simulink model "mvdc_estimation_preprocessing"  (R2018b)
settings: configuration reference "Active" (kept outside this file)
undefined symbols (not defined in the file): P_MLOC_Loc1DelayCompTime_s, P_MLOC_Loc2DelayCompTime_s, P_MLOC_OdometryManualReset_psi_rad, P_MLOC_OdometryManualReset_x_m, P_MLOC_OdometryManualReset_y_m, P_MLOC_OdometryResetMode, P_VDC_ActivateOnlineDiagnosis, P_VDC_EnableSensorsForFusion, P_VDC_SensorFailuresLatched, psi_YawAngleLoc1_rad, psi_YawAngleLoc2_rad, tS, TUMHealthStatus, TUMStateEstimationState, tw_front_m, tw_rear_m, tyreradius_front_m, tyreradius_rear_m, valid_IMU1_b, valid_IMU2_b, valid_Loc1_b, valid_Loc2_b, valid_Vel1_b, valid_Vel2_b, x_Loc1_m, x_Loc2_m, y_Loc1_m, y_Loc2_m
libraries: simulink x10, misc x6
settings Model: DataDictionary=mvdc_estimation_preprocessing.sldd  OrderedModelArguments=off  Creator=wischnewski  LastModifiedBy=ge34qer

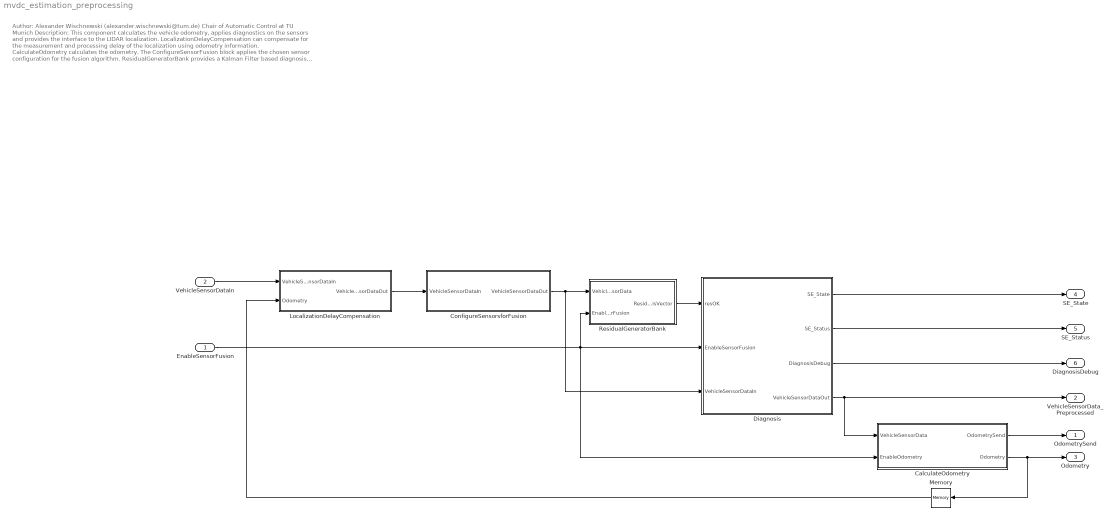
== system mvdc_estimation_preprocessing ==
  note: Author: Alexander Wischnewski (alexander.wischnewski@tum.de)
      | Chair of Automatic Control at TU Munich
      |
      | Description: This component calculates the vehicle odometry, applies diagnostics on the sensors and provides the interface to the LIDAR localization.
      |
      | LocalizationDelayCompensation can compensate for the measurement and processing delay of the localization using odometry information.
      |
      | CalculateOdometry calculates the odometry.
      |
      | The ConfigureSensorFusion block applies the chosen sensor configuration for the fusion algorithm.
      |
      | ResidualGeneratorBank provides a Kalman Filter based diagnosis on the velocity sensors. The basic idea here is to generate a fusion with one sensor missing.
      | If the Fusion without a sensor stays within the residual limits but the other does not, we know that this sensor is faulty.
      |
      | Diagnosis evaluates all the information generated and reacts accordingly.
      |
      | Inputs:
      | EnableSensorFusion Enable bit which activates the Kalman Filter
      | VehicleSensorData raw sensor data
      |
      | Outputs:
      | VisualLocSend Data which is send to the LIDAR localization algorithm
      | VehicleSensorData_Preprocessed Preprocessed data for final sensor fusion
      | Odometry Vehicle odometry as forward integrated position
      | SE_State Sensor fusion state (OK / WARNINNG / ERROR)
      | SE_Status Internal fusion mode
      | DiagnosisDebug Debug vector
  EnableSensorFusion : Inport  OutDataTypeStr=boolean  BusOutputAsStruct=on
  VehicleSensorDataIn : Inport  Port=2  OutDataTypeStr=Bus: VehicleSensorData  BusOutputAsStruct=on
  CalculateOdometry : Subsystem
  ConfigureSensorsforFusion : Subsystem
  Diagnosis : Subsystem
  LocalizationDelayCompensation : Subsystem
  Memory : Memory
  ResidualGeneratorBank : Subsystem
  OdometrySend : Outport  OutDataTypeStr=Bus: VisualLoc_Send  BusOutputAsStruct=on
  VehicleSensorData_Preprocessed : Outport  Port=2  OutDataTypeStr=Bus: VehicleSensorData  BusOutputAsStruct=on
  Odometry : Outport  Port=3  OutDataTypeStr=Bus: Odometry  BusOutputAsStruct=on
  SE_State : Outport  Port=4  OutDataTypeStr=Enum: TUMStateEstimationState
  SE_Status : Outport  Port=5  OutDataTypeStr=Enum: TUMHealthStatus
  DiagnosisDebug : Outport  Port=6  OutDataTypeStr=Bus: StateEstimation_diag
  wires:
  VehicleSensorDataIn/1 -> LocalizationDelayCompensation/1(VehicleSensorDataIn)
  LocalizationDelayCompensation/1(VehicleSensorDataOut) -> ConfigureSensorsforFusion/1(VehicleSensorDataIn)
  EnableSensorFusion/1 -> CalculateOdometry/2(EnableOdometry), Diagnosis/2(EnableSensorFusion), ResidualGeneratorBank/2(EnableSensorFusion)
  ResidualGeneratorBank/1(ResidualDiagnosisVector) -> Diagnosis/1(resOK)
  Diagnosis/1(SE_State) -> SE_State/1
  Diagnosis/2(SE_Status) -> SE_Status/1
  Diagnosis/3(DiagnosisDebug) -> DiagnosisDebug/1
  ConfigureSensorsforFusion/1(VehicleSensorDataOut) -> Diagnosis/3(VehicleSensorDataIn), ResidualGeneratorBank/1(VehicleSensorData)
  Diagnosis/4(VehicleSensorDataOut) -> CalculateOdometry/1(VehicleSensorData), VehicleSensorData_Preprocessed/1
  CalculateOdometry/2(Odometry) -> Memory/1, Odometry/1
  CalculateOdometry/1(OdometrySend) -> OdometrySend/1
  Memory/1 -> LocalizationDelayCompensation/2(Odometry)

== system mvdc_estimation_preprocessing/CalculateOdometry ==
  note: calculates an Odometry based on
      | the vehicle motion sensors. Different options are available.
      | Check "Integrate Odometry" for details.
  VehicleSensorData : Inport
  EnableOdometry : Inport  Port=2
  DetermineResetPosition : Subsystem
  ExternalOdometryInterface : Subsystem
  IntegrateOdometry : Subsystem
  OdometrySend : Outport  OutDataTypeStr=Bus: VisualLoc_Send  BusOutputAsStruct=on
  Odometry : Outport  Port=2
  wires:
  IntegrateOdometry/1(Odometry) -> ExternalOdometryInterface/1(Odometry), Odometry/1
  DetermineResetPosition/2(ResetPositionValid_b) -> ExternalOdometryInterface/3(ResetPosition_Valid), IntegrateOdometry/3(ResetPositionValid)
  DetermineResetPosition/1(ResetPosition) -> ExternalOdometryInterface/2(ResetPosition), IntegrateOdometry/2(ResetPosition)
  VehicleSensorData/1 -> ExternalOdometryInterface/4(VehicleSensorData), IntegrateOdometry/4(VehicleSensors), DetermineResetPosition/1(VehicleSensorData)
  EnableOdometry/1 -> IntegrateOdometry/1(EnableOdometry)
  ExternalOdometryInterface/1(OdometrySend) -> OdometrySend/1

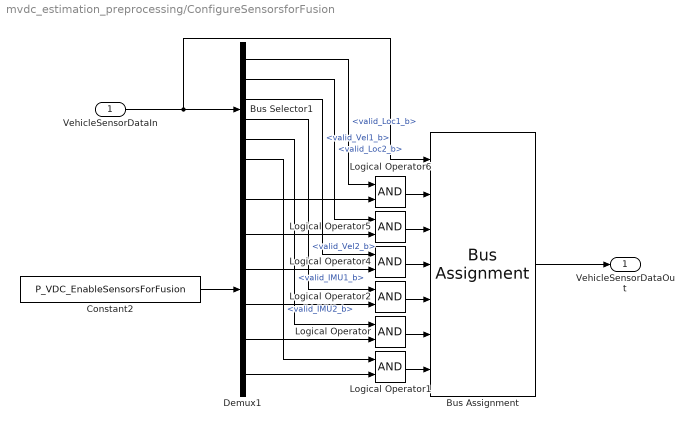
== system mvdc_estimation_preprocessing/ConfigureSensorsforFusion ==
  VehicleSensorDataIn : Inport  OutDataTypeStr=Bus: VehicleSensorData  BusOutputAsStruct=on
  Bus Assignment : BusAssignment  AssignedSignals=valid_Loc1_b,valid_Loc2_b,valid_Vel1_b,valid_Vel2_b,valid_IMU1_b,valid_IMU2_b
  Bus Selector1 : BusSelector  OutputSignals=valid_Loc1_b,valid_Loc2_b,valid_Vel1_b,valid_Vel2_b,valid_IMU1_b,valid_IMU2_b
  Constant2 : Constant  Value=P_VDC_EnableSensorsForFusion
  Demux1 : Demux  Outputs=6
  Logical Operator{,1..2,4..6} (6 alike) : Logic  AllPortsSameDT=off  OutDataTypeStr=boolean
  VehicleSensorDataOut : Outport  OutDataTypeStr=Bus: VehicleSensorData
  wires:
  Bus Assignment/1 -> VehicleSensorDataOut/1
  Demux1/6 -> Logical Operator1/2
  Bus Selector1/6 -> Logical Operator1/1  "<valid_IMU2_b>"
  Demux1/2 -> Logical Operator5/2
  Bus Selector1/4 -> Logical Operator2/1  "<valid_Vel2_b>"
  Bus Selector1/3 -> Logical Operator4/1  "<valid_Vel1_b>"
  Bus Selector1/1 -> Logical Operator6/1  "<valid_Loc1_b>"
  Constant2/1 -> Demux1/1
  Logical Operator5/1 -> Bus Assignment/3
  Logical Operator4/1 -> Bus Assignment/4
  Demux1/1 -> Logical Operator6/2
  Bus Selector1/5 -> Logical Operator/1  "<valid_IMU1_b>"
  Logical Operator/1 -> Bus Assignment/6
  Logical Operator6/1 -> Bus Assignment/2
  VehicleSensorDataIn/1 -> Bus Selector1/1, Bus Assignment/1
  Demux1/4 -> Logical Operator2/2
  Bus Selector1/2 -> Logical Operator5/1  "<valid_Loc2_b>"
  Logical Operator1/1 -> Bus Assignment/7
  Logical Operator2/1 -> Bus Assignment/5
  Demux1/3 -> Logical Operator4/2
  Demux1/5 -> Logical Operator/2

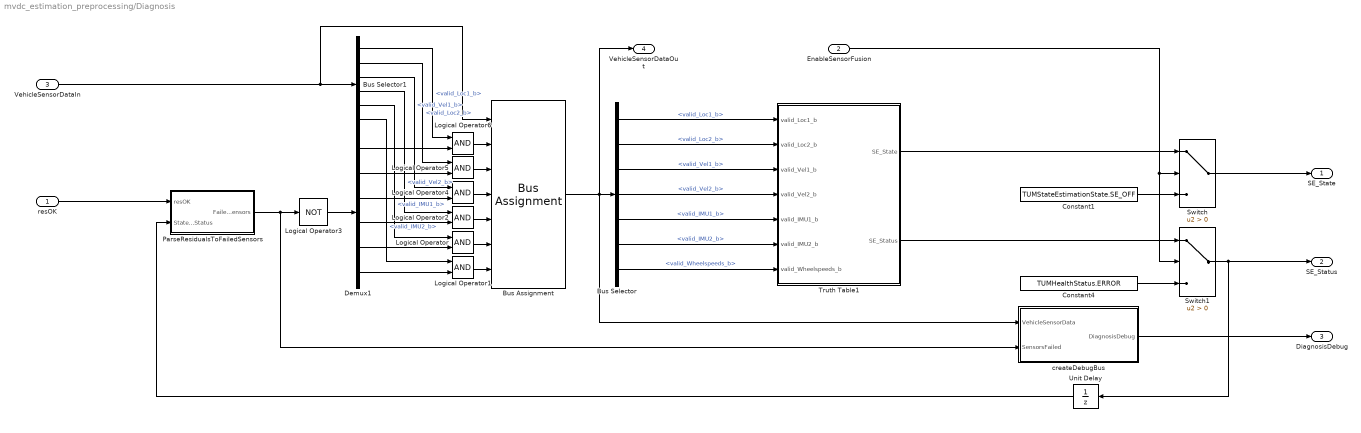
== system mvdc_estimation_preprocessing/Diagnosis ==
  resOK : Inport
  EnableSensorFusion : Inport  Port=2
  VehicleSensorDataIn : Inport  Port=3
  Bus Assignment : BusAssignment  AssignedSignals=valid_Loc1_b,valid_Loc2_b,valid_Vel1_b,valid_Vel2_b,valid_IMU1_b,valid_IMU2_b
  Bus Selector : BusSelector  OutputSignals=valid_Loc1_b,valid_Loc2_b,valid_Vel1_b,valid_Vel2_b,valid_IMU1_b,valid_IMU2_b,valid_Wheelspeeds_b
  Bus Selector1 : BusSelector  OutputSignals=valid_Loc1_b,valid_Loc2_b,valid_Vel1_b,valid_Vel2_b,valid_IMU1_b,valid_IMU2_b
  Constant1 : Constant  Value=TUMStateEstimationState.SE_OFF  OutDataTypeStr=Enum: TUMStateEstimationState
  Constant4 : Constant  Value=TUMHealthStatus.ERROR  OutDataTypeStr=Enum: TUMHealthStatus
  Demux1 : Demux  Outputs=6
  Logical Operator{,1..2,4..6} (6 alike) : Logic  AllPortsSameDT=off  OutDataTypeStr=boolean
  Logical Operator3 : Logic  Operator=NOT  Inputs=4  AllPortsSameDT=off  OutDataTypeStr=boolean
  ParseResidualsToFailedSensors : Subsystem
  Switch : Switch  Criteria=u2 > Threshold
  Switch1 : Switch  Criteria=u2 > Threshold
  Truth Table1 : Truth Table  TreatAsAtomicUnit=on
  Unit Delay : UnitDelay  InitialCondition=TUMHealthStatus.ERROR  SampleTime=-1
  createDebugBus : Subsystem
  SE_State : Outport
  SE_Status : Outport  Port=2
  DiagnosisDebug : Outport  Port=3  OutDataTypeStr=Bus: StateEstimation_diag
  VehicleSensorDataOut : Outport  Port=4
  wires:
  EnableSensorFusion/1 -> Switch1/2, Switch/2
  resOK/1 -> ParseResidualsToFailedSensors/1(resOK)
  Switch/1 -> SE_State/1
  Truth Table1/1(SE_State) -> Switch/1
  Switch1/1 -> Unit Delay/1, SE_Status/1
  Truth Table1/2(SE_Status) -> Switch1/1
  Constant1/1 -> Switch/3
  Constant4/1 -> Switch1/3
  createDebugBus/1(DiagnosisDebug) -> DiagnosisDebug/1
  ParseResidualsToFailedSensors/1(FailedSensors) -> createDebugBus/2(SensorsFailed), Logical Operator3/1
  Unit Delay/1 -> ParseResidualsToFailedSensors/2(StateEstimationStatus)
  Logical Operator3/1 -> Demux1/1
  Bus Assignment/1 -> createDebugBus/1(VehicleSensorData), VehicleSensorDataOut/1, Bus Selector/1
  Bus Selector/1 -> Truth Table1/1(valid_Loc1_b)  "<valid_Loc1_b>"
  Bus Selector/2 -> Truth Table1/2(valid_Loc2_b)  "<valid_Loc2_b>"
  Bus Selector/3 -> Truth Table1/3(valid_Vel1_b)  "<valid_Vel1_b>"
  Bus Selector/4 -> Truth Table1/4(valid_Vel2_b)  "<valid_Vel2_b>"
  Bus Selector/5 -> Truth Table1/5(valid_IMU1_b)  "<valid_IMU1_b>"
  Bus Selector/6 -> Truth Table1/6(valid_IMU2_b)  "<valid_IMU2_b>"
  Bus Selector/7 -> Truth Table1/7(valid_Wheelspeeds_b)  "<valid_Wheelspeeds_b>"
  VehicleSensorDataIn/1 -> Bus Assignment/1, Bus Selector1/1
  Logical Operator/1 -> Bus Assignment/6
  Logical Operator1/1 -> Bus Assignment/7
  Logical Operator2/1 -> Bus Assignment/5
  Logical Operator4/1 -> Bus Assignment/4
  Logical Operator6/1 -> Bus Assignment/2
  Logical Operator5/1 -> Bus Assignment/3
  Demux1/6 -> Logical Operator1/2
  Demux1/5 -> Logical Operator/2
  Demux1/4 -> Logical Operator2/2
  Demux1/3 -> Logical Operator4/2
  Demux1/2 -> Logical Operator5/2
  Demux1/1 -> Logical Operator6/2
  Bus Selector1/6 -> Logical Operator1/1  "<valid_IMU2_b>"
  Bus Selector1/5 -> Logical Operator/1  "<valid_IMU1_b>"
  Bus Selector1/4 -> Logical Operator2/1  "<valid_Vel2_b>"
  Bus Selector1/3 -> Logical Operator4/1  "<valid_Vel1_b>"
  Bus Selector1/2 -> Logical Operator5/1  "<valid_Loc2_b>"
  Bus Selector1/1 -> Logical Operator6/1  "<valid_Loc1_b>"

== system mvdc_estimation_preprocessing/LocalizationDelayCompensation ==
  VehicleSensorDataIn : Inport
  Odometry : Inport  Port=2  OutDataTypeStr=Bus: Odometry
  Bus Assignment : BusAssignment  AssignedSignals=x_Loc1_m,y_Loc1_m,psi_YawAngleLoc1_rad,valid_Loc1_b,x_Loc2_m,y_Loc2_m,psi_YawAngleLoc2_rad,valid_Loc2_b
  Bus Selector : BusSelector  OutputSignals=x_Loc1_m,y_Loc1_m,psi_YawAngleLoc1_rad,valid_Loc1_b
  Bus Selector1 : BusSelector  OutputSignals=x_Loc2_m,y_Loc2_m,psi_YawAngleLoc2_rad,valid_Loc2_b
  CompensateLocaliization2 : Subsystem
  CompensateLocalization1 : Subsystem
  VehicleSensorDataOut : Outport
  wires:
  VehicleSensorDataIn/1 -> CompensateLocaliization2/1(VehicleSensorData), CompensateLocalization1/1(VehicleSensorData), Bus Assignment/1
  Bus Assignment/1 -> VehicleSensorDataOut/1
  Odometry/1 -> CompensateLocaliization2/2(Odometry), CompensateLocalization1/2(Odometry)
  CompensateLocalization1/1(Loc1Comp) -> Bus Selector/1
  Bus Selector/1 -> Bus Assignment/2  "<x_Loc1_m>"
  Bus Selector/2 -> Bus Assignment/3  "<y_Loc1_m>"
  Bus Selector/3 -> Bus Assignment/4  "<psi_YawAngleLoc1_rad>"
  Bus Selector/4 -> Bus Assignment/5  "<valid_Loc1_b>"
  CompensateLocaliization2/1(Loc2Comp) -> Bus Selector1/1
  Bus Selector1/1 -> Bus Assignment/6  "<x_Loc2_m>"
  Bus Selector1/2 -> Bus Assignment/7  "<y_Loc2_m>"
  Bus Selector1/3 -> Bus Assignment/8  "<psi_YawAngleLoc2_rad>"
  Bus Selector1/4 -> Bus Assignment/9  "<valid_Loc2_b>"

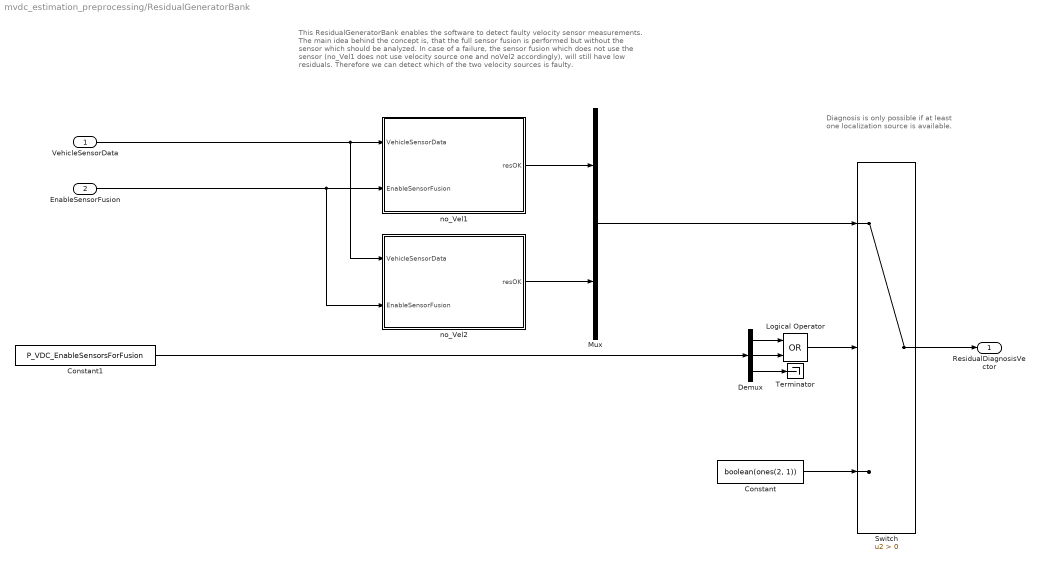
== system mvdc_estimation_preprocessing/ResidualGeneratorBank ==
  note: This ResidualGeneratorBank enables the software to detect faulty
      | velocity sensor measurements. The main idea behind the concept is,
      | that the full sensor fusion is performed but without the sensor which should be analyzed.
      | In case of a failure, the sensor fusion which does not use the sensor (no_Vel1 does not use
      | velocity source one and noVel2 accordingly), will still have low residuals. Therefore
      | we can detect which of the two velocity sources is faulty.
  note: Diagnosis is only possible if at least
      | one localization source is available.
  VehicleSensorData : Inport
  EnableSensorFusion : Inport  Port=2
  Constant : Constant  Value=boolean(ones(2, 1))
  Constant1 : Constant  Value=P_VDC_EnableSensorsForFusion
  Demux : Demux  Outputs=[1 1 4]
  Logical Operator : Logic  Operator=OR  AllPortsSameDT=off  OutDataTypeStr=boolean
  Mux : Mux  Inputs=2
  Switch : Switch  Criteria=u2 > Threshold
  Terminator : Terminator
  no_Vel1 : Subsystem
  no_Vel2 : Subsystem
  ResidualDiagnosisVector : Outport
  wires:
  VehicleSensorData/1 -> no_Vel1/1(VehicleSensorData), no_Vel2/1(VehicleSensorData)
  EnableSensorFusion/1 -> no_Vel1/2(EnableSensorFusion), no_Vel2/2(EnableSensorFusion)
  Constant1/1 -> Demux/1
  Mux/1 -> Switch/1
  Switch/1 -> ResidualDiagnosisVector/1
  Constant/1 -> Switch/3
  Logical Operator/1 -> Switch/2
  Demux/2 -> Logical Operator/2
  Demux/1 -> Logical Operator/1
  Demux/3 -> Terminator/1
  no_Vel1/1(resOK) -> Mux/1
  no_Vel2/1(resOK) -> Mux/2

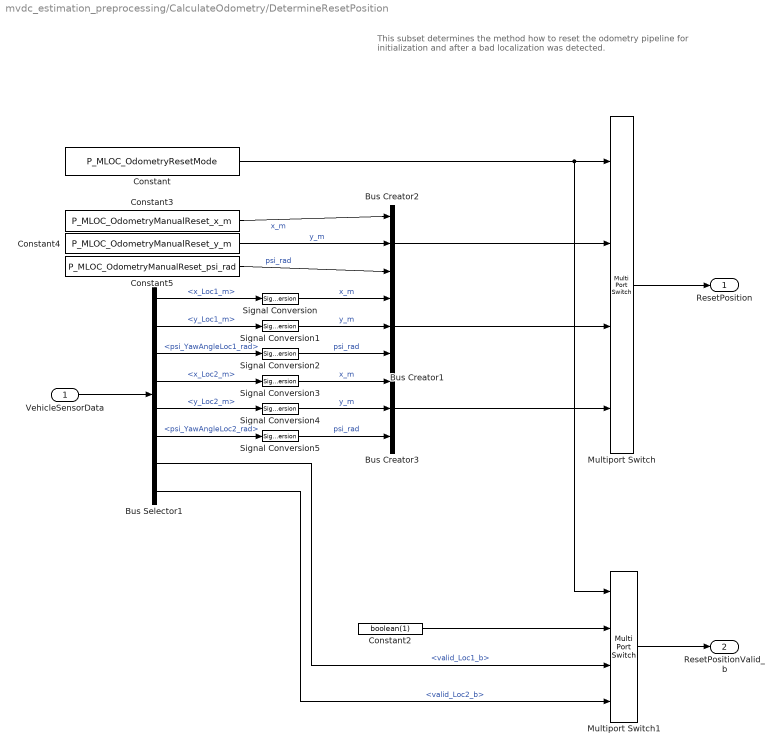
== system mvdc_estimation_preprocessing/CalculateOdometry/DetermineResetPosition ==
  note: This subset determines the method how to reset the
      | odometry pipeline for initialization and after a bad localization was detected.
  VehicleSensorData : Inport
  Bus Creator1 : BusCreator  Inputs=3  OutDataTypeStr=Bus: CartPos
  Bus Creator2 : BusCreator  Inputs=3  OutDataTypeStr=Bus: CartPos
  Bus Creator3 : BusCreator  Inputs=3  OutDataTypeStr=Bus: CartPos
  Bus Selector1 : BusSelector  OutputSignals=x_Loc1_m,y_Loc1_m,psi_YawAngleLoc1_rad,x_Loc2_m,y_Loc2_m,psi_YawAngleLoc2_rad,valid_Loc1_b,valid_Loc2_b
  Constant : Constant  Value=P_MLOC_OdometryResetMode
  Constant2 : Constant  Value=boolean(1)
  Constant3 : Constant  Value=P_MLOC_OdometryManualReset_x_m
  Constant4 : Constant  Value=P_MLOC_OdometryManualReset_y_m
  Constant5 : Constant  Value=P_MLOC_OdometryManualReset_psi_rad
  Multiport Switch : MultiPortSwitch
  Multiport Switch1 : MultiPortSwitch
  Signal Conversion{,1..5} (6 alike) : SignalConversion  OverrideOpt=off
  ResetPosition : Outport
  ResetPositionValid_b : Outport  Port=2
  wires:
  Constant3/1 -> Bus Creator2/1  "x_m"
  Constant4/1 -> Bus Creator2/2  "y_m"
  Constant5/1 -> Bus Creator2/3  "psi_rad"
  Bus Creator2/1 -> Multiport Switch/2
  VehicleSensorData/1 -> Bus Selector1/1
  Signal Conversion/1 -> Bus Creator1/1  "x_m"
  Bus Selector1/1 -> Signal Conversion/1  "<x_Loc1_m>"
  Bus Selector1/2 -> Signal Conversion1/1  "<y_Loc1_m>"
  Bus Selector1/3 -> Signal Conversion2/1  "<psi_YawAngleLoc1_rad>"
  Signal Conversion2/1 -> Bus Creator1/3  "psi_rad"
  Signal Conversion1/1 -> Bus Creator1/2  "y_m"
  Bus Creator1/1 -> Multiport Switch/3
  Multiport Switch/1 -> ResetPosition/1
  Multiport Switch1/1 -> ResetPositionValid_b/1
  Constant2/1 -> Multiport Switch1/2
  Bus Selector1/7 -> Multiport Switch1/3  "<valid_Loc1_b>"
  Constant/1 -> Multiport Switch1/1, Multiport Switch/1
  Bus Selector1/4 -> Signal Conversion3/1  "<x_Loc2_m>"
  Bus Selector1/5 -> Signal Conversion4/1  "<y_Loc2_m>"
  Bus Selector1/6 -> Signal Conversion5/1  "<psi_YawAngleLoc2_rad>"
  Bus Selector1/8 -> Multiport Switch1/4  "<valid_Loc2_b>"
  Signal Conversion3/1 -> Bus Creator3/1  "x_m"
  Signal Conversion4/1 -> Bus Creator3/2  "y_m"
  Signal Conversion5/1 -> Bus Creator3/3  "psi_rad"
  Bus Creator3/1 -> Multiport Switch/4

== system mvdc_estimation_preprocessing/CalculateOdometry/ExternalOdometryInterface ==
  Odometry : Inport
  ResetPosition : Inport  Port=2
  ResetPosition_Valid : Inport  Port=3
  VehicleSensorData : Inport  Port=4
  Bus Creator : BusCreator  Inputs=7
  Bus Selector : BusSelector  OutputSignals=t_EstimateLoc1_s,vx_CoGVel1_mps,vy_CoGVel1_mps,dPsi_YawRateIMU1_radps
  Signal Conversion{1..4} (4 alike) : SignalConversion  OverrideOpt=off
  OdometrySend : Outport  BusOutputAsStruct=on
  wires:
  Bus Creator/1 -> OdometrySend/1
  VehicleSensorData/1 -> Bus Selector/1
  Bus Selector/1 -> Signal Conversion4/1  "<t_EstimateLoc1_s>"
  Signal Conversion4/1 -> Bus Creator/1  "timeGPS_s"
  Bus Selector/2 -> Signal Conversion1/1  "<vx_CoGVel1_mps>"
  Bus Selector/3 -> Signal Conversion2/1  "<vy_CoGVel1_mps>"
  Bus Selector/4 -> Signal Conversion3/1  "<dPsi_YawRateIMU1_radps>"
  ResetPosition/1 -> Bus Creator/5  "ResetPosition"
  ResetPosition_Valid/1 -> Bus Creator/6  "ResetPosition_Valid"
  Odometry/1 -> Bus Creator/7  "Odometry"
  Signal Conversion1/1 -> Bus Creator/2  "vx_mps"
  Signal Conversion2/1 -> Bus Creator/3  "vy_mps"
  Signal Conversion3/1 -> Bus Creator/4  "dPsi_radps"

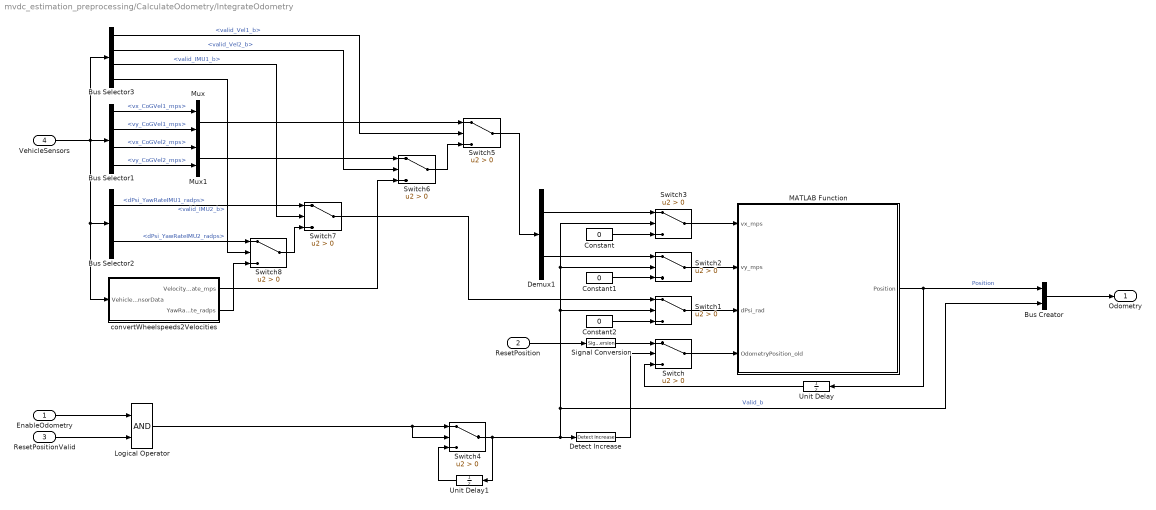
== system mvdc_estimation_preprocessing/CalculateOdometry/IntegrateOdometry ==
  EnableOdometry : Inport
  ResetPosition : Inport  Port=2
  ResetPositionValid : Inport  Port=3
  VehicleSensors : Inport  Port=4
  Bus Creator : BusCreator  Inputs=2
  Bus Selector1 : BusSelector  OutputSignals=vx_CoGVel1_mps,vy_CoGVel1_mps,vx_CoGVel2_mps,vy_CoGVel2_mps
  Bus Selector2 : BusSelector  OutputSignals=dPsi_YawRateIMU1_radps,dPsi_YawRateIMU2_radps
  Bus Selector3 : BusSelector  OutputSignals=valid_Vel1_b,valid_Vel2_b,valid_IMU1_b,valid_IMU2_b
  Constant : Constant  Value=0
  Constant1 : Constant  Value=0
  Constant2 : Constant  Value=0
  Demux1 : Demux  Outputs=2
  Detect Increase : simulink/Logic and Bit Operations/Detect Increase  vinit=0.0  OutDataTypeStr=boolean
  Logical Operator : Logic  AllPortsSameDT=off  OutDataTypeStr=boolean
  MATLAB Function : MATLAB Function  TreatAsAtomicUnit=on
  Mux : Mux  Inputs=2
  Mux1 : Mux  Inputs=2
  Signal Conversion : SignalConversion  ConversionOutput=Nonvirtual bus  OverrideOpt=off
  Switch{,1..8} (9 alike) : Switch  Criteria=u2 > Threshold
  Unit Delay : UnitDelay  SampleTime=-1
  Unit Delay1 : UnitDelay  SampleTime=-1
  convertWheelspeeds2Velocities : Subsystem
  Odometry : Outport  BusOutputAsStruct=on
  wires:
  Switch/1 -> MATLAB Function/4(OdometryPosition_old)
  Unit Delay/1 -> Switch/3
  Switch1/1 -> MATLAB Function/3(dPsi_rad)
  Switch2/1 -> MATLAB Function/2(vy_mps)
  Switch3/1 -> MATLAB Function/1(vx_mps)
  Constant/1 -> Switch3/3
  Constant1/1 -> Switch2/3
  Constant2/1 -> Switch1/3
  Logical Operator/1 -> Switch4/2, Switch4/1
  Unit Delay1/1 -> Switch4/3
  Switch4/1 -> Detect Increase/1, Bus Creator/2, Switch3/2, Switch2/2, Switch1/2, Unit Delay1/1  "Valid_b"
  Detect Increase/1 -> Switch/2
  MATLAB Function/1(Position) -> Unit Delay/1, Bus Creator/1  "Position"
  Bus Creator/1 -> Odometry/1
  VehicleSensors/1 -> convertWheelspeeds2Velocities/1(VehicleSensorData), Bus Selector2/1, Bus Selector3/1, Bus Selector1/1
  EnableOdometry/1 -> Logical Operator/1
  ResetPositionValid/1 -> Logical Operator/2
  Signal Conversion/1 -> Switch/1
  ResetPosition/1 -> Signal Conversion/1
  Bus Selector1/1 -> Mux/1  "<vx_CoGVel1_mps>"
  Bus Selector1/2 -> Mux/2  "<vy_CoGVel1_mps>"
  Bus Selector1/3 -> Mux1/1  "<vx_CoGVel2_mps>"
  Bus Selector1/4 -> Mux1/2  "<vy_CoGVel2_mps>"
  Mux/1 -> Switch5/1
  Switch6/1 -> Switch5/3
  Mux1/1 -> Switch6/1
  convertWheelspeeds2Velocities/1(VelocityEstimate_mps) -> Switch6/3
  Bus Selector2/1 -> Switch7/1  "<dPsi_YawRateIMU1_radps>"
  Bus Selector2/2 -> Switch8/1  "<dPsi_YawRateIMU2_radps>"
  Switch8/1 -> Switch7/3
  convertWheelspeeds2Velocities/2(YawRateEstimate_radps) -> Switch8/3
  Switch7/1 -> Switch1/1
  Demux1/1 -> Switch3/1
  Demux1/2 -> Switch2/1
  Switch5/1 -> Demux1/1
  Bus Selector3/1 -> Switch5/2  "<valid_Vel1_b>"
  Bus Selector3/2 -> Switch6/2  "<valid_Vel2_b>"
  Bus Selector3/3 -> Switch7/2  "<valid_IMU1_b>"
  Bus Selector3/4 -> Switch8/2  "<valid_IMU2_b>"

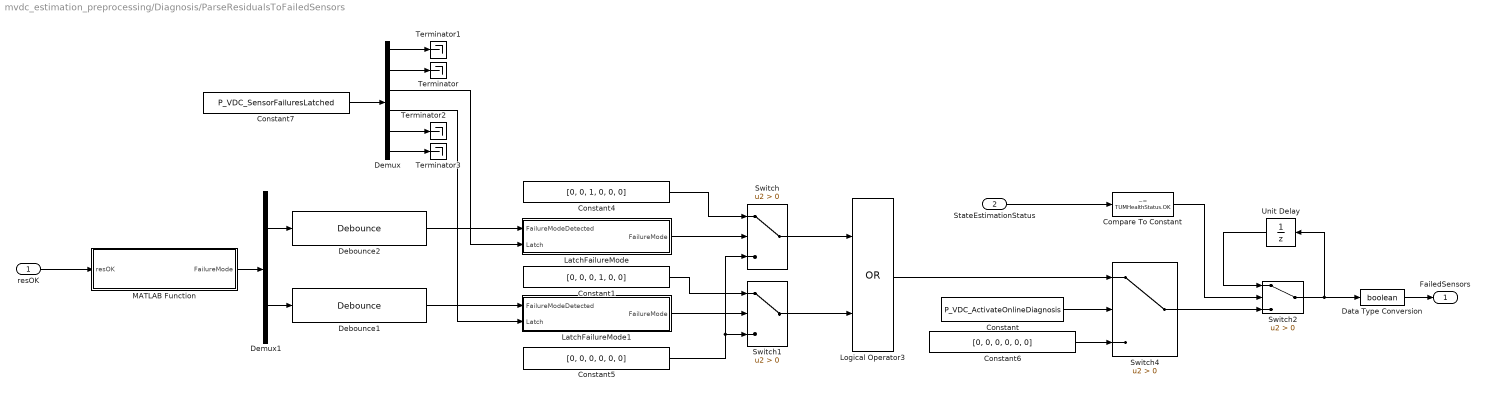
== system mvdc_estimation_preprocessing/Diagnosis/ParseResidualsToFailedSensors ==
  resOK : Inport
  StateEstimationStatus : Inport  Port=2
  Compare To Constant : simulink/Logic and Bit Operations/Compare To Constant  relop=~=  const=TUMHealthStatus.OK  OutDataTypeStr=boolean
  Constant : Constant  Value=P_VDC_ActivateOnlineDiagnosis
  Constant1 : Constant  Value=[0, 0, 0, 1, 0, 0]
  Constant4 : Constant  Value=[0, 0, 1, 0, 0, 0]
  Constant5 : Constant  Value=[0, 0, 0, 0, 0, 0]
  Constant6 : Constant  Value=[0, 0, 0, 0, 0, 0]
  Constant7 : Constant  Value=P_VDC_SensorFailuresLatched
  Data Type Conversion : DataTypeConversion  OutDataTypeStr=boolean
  Debounce1 : misc/Debounce  debounce_cycles=P_VDC_DebounceSensorFailure
  Debounce2 : misc/Debounce  debounce_cycles=P_VDC_DebounceSensorFailure
  Demux : Demux  Outputs=6
  Demux1 : Demux  Outputs=2
  LatchFailureMode : Subsystem
  LatchFailureMode1 : Subsystem
  Logical Operator3 : Logic  Operator=OR  AllPortsSameDT=off  OutDataTypeStr=boolean
  MATLAB Function : MATLAB Function  TreatAsAtomicUnit=on
  Switch{,1..2,4} (4 alike) : Switch  Criteria=u2 > Threshold
  Terminator{,1..3} (4 alike) : Terminator
  Unit Delay : UnitDelay  SampleTime=-1
  FailedSensors : Outport
  wires:
  Switch1/1 -> Logical Operator3/2
  Constant4/1 -> Switch/1
  LatchFailureMode1/1(FailureMode) -> Switch1/2
  Constant5/1 -> Switch1/3, Switch/3
  MATLAB Function/1(FailureMode) -> Demux1/1
  Demux1/1 -> Debounce2/1
  Switch/1 -> Logical Operator3/1
  LatchFailureMode/1(FailureMode) -> Switch/2
  Constant1/1 -> Switch1/1
  resOK/1 -> MATLAB Function/1(resOK)
  Demux1/2 -> Debounce1/1
  Debounce2/1 -> LatchFailureMode/1(FailureModeDetected)
  Debounce1/1 -> LatchFailureMode1/1(FailureModeDetected)
  Constant/1 -> Switch4/2
  Logical Operator3/1 -> Switch4/1
  Constant6/1 -> Switch4/3
  Constant7/1 -> Demux/1
  Demux/4 -> LatchFailureMode1/2(Latch)
  Demux/3 -> LatchFailureMode/2(Latch)
  Demux/2 -> Terminator/1
  Demux/1 -> Terminator1/1
  Demux/5 -> Terminator2/1
  Demux/6 -> Terminator3/1
  Switch4/1 -> Switch2/3
  Switch2/1 -> Unit Delay/1, Data Type Conversion/1
  Unit Delay/1 -> Switch2/1
  Data Type Conversion/1 -> FailedSensors/1
  StateEstimationStatus/1 -> Compare To Constant/1
  Compare To Constant/1 -> Switch2/2

== system mvdc_estimation_preprocessing/Diagnosis/createDebugBus ==
  VehicleSensorData : Inport
  SensorsFailed : Inport  Port=2
  Bus Creator : BusCreator  Inputs=12
  Bus Selector : BusSelector  OutputSignals=valid_Loc1_b,valid_Loc2_b,valid_Vel1_b,valid_Vel2_b,valid_IMU1_b,valid_IMU2_b
  Demux2 : Demux  Outputs=6
  DiagnosisDebug : Outport
  wires:
  Bus Selector/5 -> Bus Creator/5  "<valid_IMU1_b>"
  Bus Selector/1 -> Bus Creator/1  "<valid_Loc1_b>"
  Bus Selector/6 -> Bus Creator/6  "<valid_IMU2_b>"
  Bus Selector/2 -> Bus Creator/2  "<valid_Loc2_b>"
  Bus Selector/3 -> Bus Creator/3  "<valid_Vel1_b>"
  Bus Selector/4 -> Bus Creator/4  "<valid_Vel2_b>"
  SensorsFailed/1 -> Demux2/1
  VehicleSensorData/1 -> Bus Selector/1
  Bus Creator/1 -> DiagnosisDebug/1
  Demux2/1 -> Bus Creator/7  "fail_Loc1_b"
  Demux2/2 -> Bus Creator/8  "fail_Loc2_b"
  Demux2/3 -> Bus Creator/9  "fail_Vel1_b"
  Demux2/4 -> Bus Creator/10  "fail_Vel2_b"
  Demux2/5 -> Bus Creator/11  "fail_IMU1_b"
  Demux2/6 -> Bus Creator/12  "fail_IMU2_b"

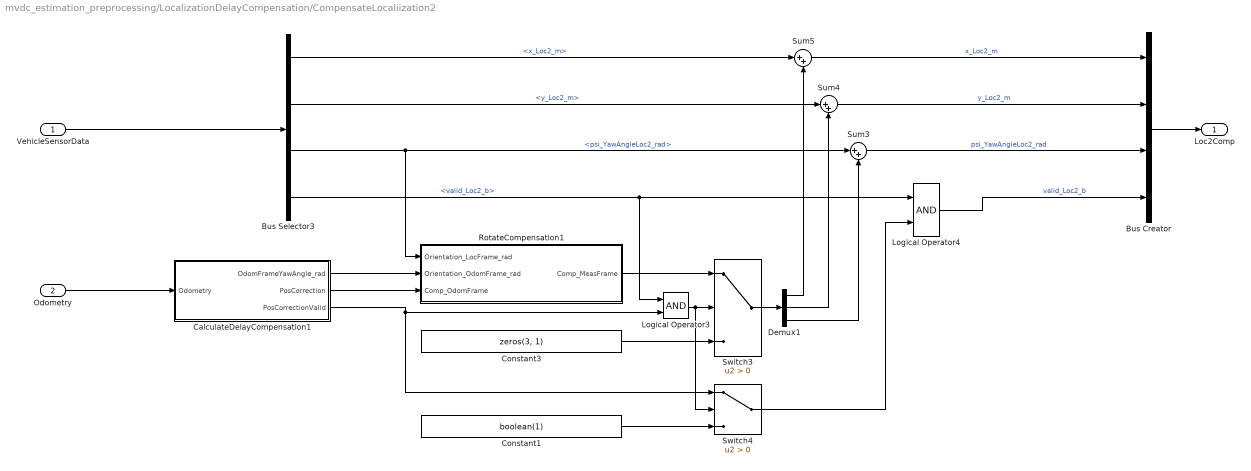
== system mvdc_estimation_preprocessing/LocalizationDelayCompensation/CompensateLocaliization2 ==
  VehicleSensorData : Inport
  Odometry : Inport  Port=2
  Bus Creator : BusCreator  Inputs=4
  Bus Selector3 : BusSelector  OutputSignals=x_Loc2_m,y_Loc2_m,psi_YawAngleLoc2_rad,valid_Loc2_b
  CalculateDelayCompensation1 : Subsystem
  Constant1 : Constant  Value=boolean(1)
  Constant3 : Constant  Value=zeros(3, 1)
  Demux1 : Demux  Outputs=3
  Logical Operator3 : Logic  AllPortsSameDT=off  OutDataTypeStr=boolean
  Logical Operator4 : Logic  AllPortsSameDT=off  OutDataTypeStr=boolean
  RotateCompensation1 : Subsystem
  Sum3 : Sum  Inputs=|++
  Sum4 : Sum  Inputs=|++
  Sum5 : Sum  Inputs=|++
  Switch3 : Switch  Criteria=u2 > Threshold
  Switch4 : Switch  Criteria=u2 > Threshold
  Loc2Comp : Outport
  wires:
  Logical Operator3/1 -> Switch4/2, Switch3/2
  Switch4/1 -> Logical Operator4/2
  Bus Selector3/4 -> Logical Operator4/1, Logical Operator3/1  "<valid_Loc2_b>"
  Demux1/3 -> Sum3/2
  Demux1/2 -> Sum4/2
  Switch3/1 -> Demux1/1
  RotateCompensation1/1(Comp_MeasFrame) -> Switch3/1
  CalculateDelayCompensation1/2(PosCorrection) -> RotateCompensation1/3(Comp_OdomFrame)
  Odometry/1 -> CalculateDelayCompensation1/1(Odometry)
  Bus Selector3/1 -> Sum5/1  "<x_Loc2_m>"
  CalculateDelayCompensation1/3(PosCorrectionValid) -> Switch4/1, Logical Operator3/2
  Bus Selector3/2 -> Sum4/1  "<y_Loc2_m>"
  Bus Selector3/3 -> Sum3/1, RotateCompensation1/1(Orientation_LocFrame_rad)  "<psi_YawAngleLoc2_rad>"
  Constant3/1 -> Switch3/3
  VehicleSensorData/1 -> Bus Selector3/1
  Constant1/1 -> Switch4/3
  Demux1/1 -> Sum5/2
  Sum5/1 -> Bus Creator/1  "x_Loc2_m"
  Sum4/1 -> Bus Creator/2  "y_Loc2_m"
  Sum3/1 -> Bus Creator/3  "psi_YawAngleLoc2_rad"
  Logical Operator4/1 -> Bus Creator/4  "valid_Loc2_b"
  Bus Creator/1 -> Loc2Comp/1
  CalculateDelayCompensation1/1(OdomFrameYawAngle_rad) -> RotateCompensation1/2(Orientation_OdomFrame_rad)

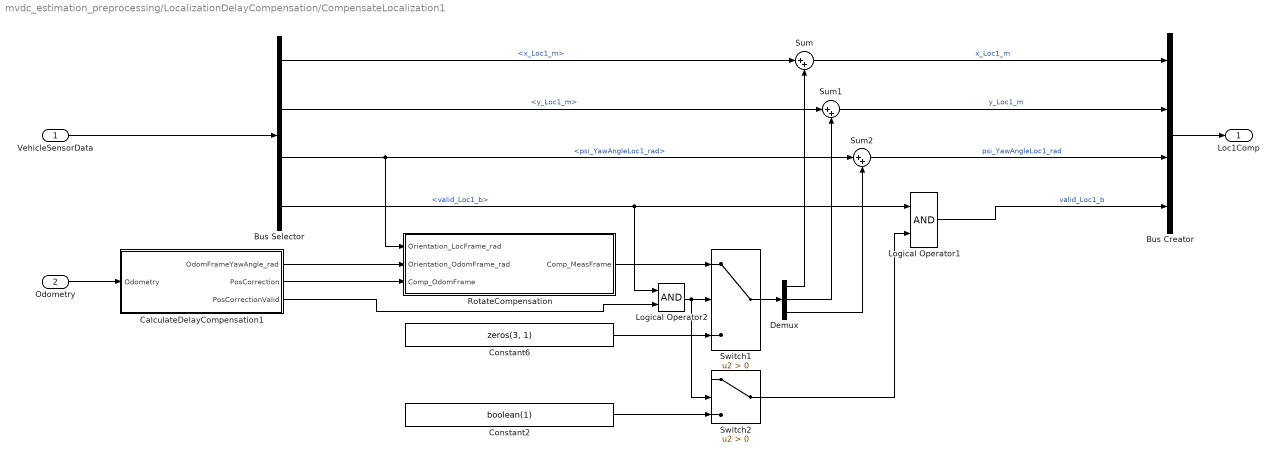
== system mvdc_estimation_preprocessing/LocalizationDelayCompensation/CompensateLocalization1 ==
  VehicleSensorData : Inport
  Odometry : Inport  Port=2
  Bus Creator : BusCreator  Inputs=4
  Bus Selector : BusSelector  OutputSignals=x_Loc1_m,y_Loc1_m,psi_YawAngleLoc1_rad,valid_Loc1_b
  CalculateDelayCompensation1 : Subsystem
  Constant2 : Constant  Value=boolean(1)
  Constant6 : Constant  Value=zeros(3, 1)
  Demux : Demux  Outputs=3
  Logical Operator1 : Logic  AllPortsSameDT=off  OutDataTypeStr=boolean
  Logical Operator2 : Logic  AllPortsSameDT=off  OutDataTypeStr=boolean
  RotateCompensation : Subsystem
  Sum : Sum  Inputs=|++
  Sum1 : Sum  Inputs=|++
  Sum2 : Sum  Inputs=|++
  Switch1 : Switch  Criteria=u2 > Threshold
  Switch2 : Switch  Criteria=u2 > Threshold
  Loc1Comp : Outport
  wires:
  Bus Selector/4 -> Logical Operator2/1, Logical Operator1/1  "<valid_Loc1_b>"
  Logical Operator2/1 -> Switch2/2, Switch1/2
  Switch2/1 -> Logical Operator1/2
  Bus Selector/2 -> Sum1/1  "<y_Loc1_m>"
  CalculateDelayCompensation1/1(OdomFrameYawAngle_rad) -> RotateCompensation/2(Orientation_OdomFrame_rad)
  Bus Selector/3 -> RotateCompensation/1(Orientation_LocFrame_rad), Sum2/1  "<psi_YawAngleLoc1_rad>"
  Demux/2 -> Sum1/2
  Bus Selector/1 -> Sum/1  "<x_Loc1_m>"
  Constant6/1 -> Switch1/3
  Constant2/1 -> Switch2/3
  Demux/1 -> Sum/2
  Demux/3 -> Sum2/2
  Switch1/1 -> Demux/1
  RotateCompensation/1(Comp_MeasFrame) -> Switch1/1
  Odometry/1 -> CalculateDelayCompensation1/1(Odometry)
  VehicleSensorData/1 -> Bus Selector/1
  Logical Operator1/1 -> Bus Creator/4  "valid_Loc1_b"
  Sum2/1 -> Bus Creator/3  "psi_YawAngleLoc1_rad"
  Sum1/1 -> Bus Creator/2  "y_Loc1_m"
  Sum/1 -> Bus Creator/1  "x_Loc1_m"
  Bus Creator/1 -> Loc1Comp/1
  CalculateDelayCompensation1/2(PosCorrection) -> RotateCompensation/3(Comp_OdomFrame)
  CalculateDelayCompensation1/3(PosCorrectionValid) -> Logical Operator2/2

== system mvdc_estimation_preprocessing/ResidualGeneratorBank/no_Vel1 ==
  VehicleSensorData : Inport
  EnableSensorFusion : Inport  Port=2
  Bus Assignment : BusAssignment  AssignedSignals=valid_Vel1_b
  Constant : Constant  Value=boolean(0)
  Terminator : Terminator
  Terminator1 : Terminator
  mvdc_KF_PointMassJoint.slx : ModelReference  ModelNameDialog=mvdc_KF_PointMassJoint.slx  SimulationMode=Normal  ModelReferenceVersion=1.174
  resOK : Outport
  wires:
  mvdc_KF_PointMassJoint.slx/1 -> Terminator/1
  mvdc_KF_PointMassJoint.slx/3 -> resOK/1
  EnableSensorFusion/1 -> mvdc_KF_PointMassJoint.slx/1
  mvdc_KF_PointMassJoint.slx/2 -> Terminator1/1
  VehicleSensorData/1 -> Bus Assignment/1
  Bus Assignment/1 -> mvdc_KF_PointMassJoint.slx/2
  Constant/1 -> Bus Assignment/2

== system mvdc_estimation_preprocessing/ResidualGeneratorBank/no_Vel2 ==
  VehicleSensorData : Inport
  EnableSensorFusion : Inport  Port=2
  Bus Assignment : BusAssignment  AssignedSignals=valid_Vel2_b
  Constant : Constant  Value=boolean(0)
  Terminator : Terminator
  Terminator1 : Terminator
  mvdc_KF_PointMassJoint.slx : ModelReference  ModelNameDialog=mvdc_KF_PointMassJoint.slx  SimulationMode=Normal  ModelReferenceVersion=1.174
  resOK : Outport
  wires:
  mvdc_KF_PointMassJoint.slx/1 -> Terminator/1
  mvdc_KF_PointMassJoint.slx/3 -> resOK/1
  EnableSensorFusion/1 -> mvdc_KF_PointMassJoint.slx/1
  Constant/1 -> Bus Assignment/2
  VehicleSensorData/1 -> Bus Assignment/1
  Bus Assignment/1 -> mvdc_KF_PointMassJoint.slx/2
  mvdc_KF_PointMassJoint.slx/2 -> Terminator1/1

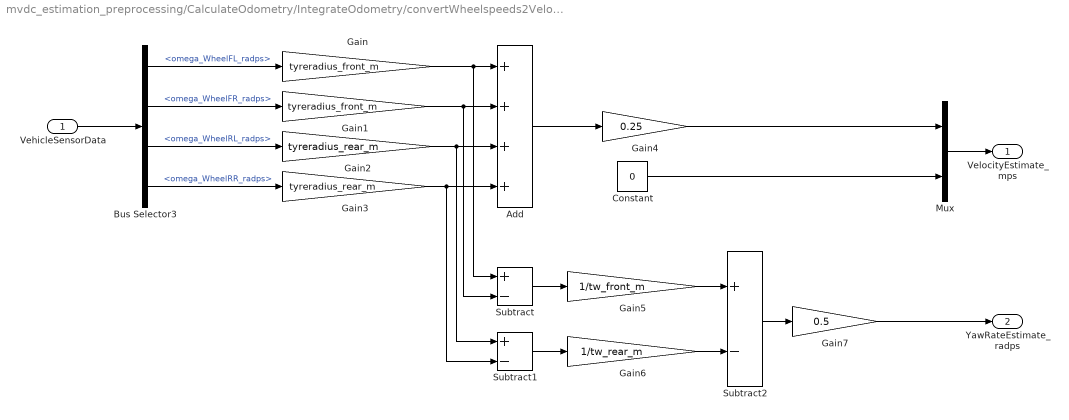
== system mvdc_estimation_preprocessing/CalculateOdometry/IntegrateOdometry/convertWheelspeeds2Velocities ==
  VehicleSensorData : Inport
  Add : Sum  Inputs=4
  Bus Selector3 : BusSelector  OutputSignals=omega_WheelFL_radps,omega_WheelFR_radps,omega_WheelRL_radps,omega_WheelRR_radps
  Constant : Constant  Value=0
  Gain : Gain  Gain=tyreradius_front_m
  Gain1 : Gain  Gain=tyreradius_front_m
  Gain2 : Gain  Gain=tyreradius_rear_m
  Gain3 : Gain  Gain=tyreradius_rear_m
  Gain4 : Gain  Gain=0.25
  Gain5 : Gain  Gain=1/tw_front_m
  Gain6 : Gain  Gain=1/tw_rear_m
  Gain7 : Gain  Gain=0.5
  Mux : Mux  Inputs=2
  Subtract : Sum  Inputs=+-
  Subtract1 : Sum  Inputs=+-
  Subtract2 : Sum  Inputs=+-
  VelocityEstimate_mps : Outport
  YawRateEstimate_radps : Outport  Port=2
  wires:
  Gain2/1 -> Subtract1/1, Add/3
  Gain/1 -> Subtract/1, Add/1
  Bus Selector3/3 -> Gain2/1  "<omega_WheelRL_radps>"
  VehicleSensorData/1 -> Bus Selector3/1
  Gain1/1 -> Subtract/2, Add/2
  Bus Selector3/4 -> Gain3/1  "<omega_WheelRR_radps>"
  Bus Selector3/1 -> Gain/1  "<omega_WheelFL_radps>"
  Bus Selector3/2 -> Gain1/1  "<omega_WheelFR_radps>"
  Gain3/1 -> Subtract1/2, Add/4
  Add/1 -> Gain4/1
  Gain4/1 -> Mux/1
  Constant/1 -> Mux/2
  Mux/1 -> VelocityEstimate_mps/1
  Subtract/1 -> Gain5/1
  Subtract1/1 -> Gain6/1
  Gain5/1 -> Subtract2/1
  Gain6/1 -> Subtract2/2
  Subtract2/1 -> Gain7/1
  Gain7/1 -> YawRateEstimate_radps/1

== system mvdc_estimation_preprocessing/Diagnosis/ParseResidualsToFailedSensors/LatchFailureMode ==
  FailureModeDetected : Inport
  Latch : Inport  Port=2
  Constant1 : Constant  Value=boolean(1)
  Delay2 : Delay  DelayLength=1  InitialCondition=0
  Switch : Switch  Criteria=u2 > Threshold
  Switch1 : Switch  Criteria=u2 > Threshold
  FailureMode : Outport
  wires:
  FailureModeDetected/1 -> Switch1/3, Switch/2
  Switch/1 -> Delay2/1
  Constant1/1 -> Switch/1
  Delay2/1 -> Switch/3, Switch1/1
  Latch/1 -> Switch1/2
  Switch1/1 -> FailureMode/1

== system mvdc_estimation_preprocessing/Diagnosis/ParseResidualsToFailedSensors/LatchFailureMode1 ==
  FailureModeDetected : Inport
  Latch : Inport  Port=2
  Constant1 : Constant  Value=boolean(1)
  Delay2 : Delay  DelayLength=1  InitialCondition=0
  Switch : Switch  Criteria=u2 > Threshold
  Switch1 : Switch  Criteria=u2 > Threshold
  FailureMode : Outport
  wires:
  FailureModeDetected/1 -> Switch1/3, Switch/2
  Switch/1 -> Delay2/1
  Constant1/1 -> Switch/1
  Delay2/1 -> Switch/3, Switch1/1
  Latch/1 -> Switch1/2
  Switch1/1 -> FailureMode/1

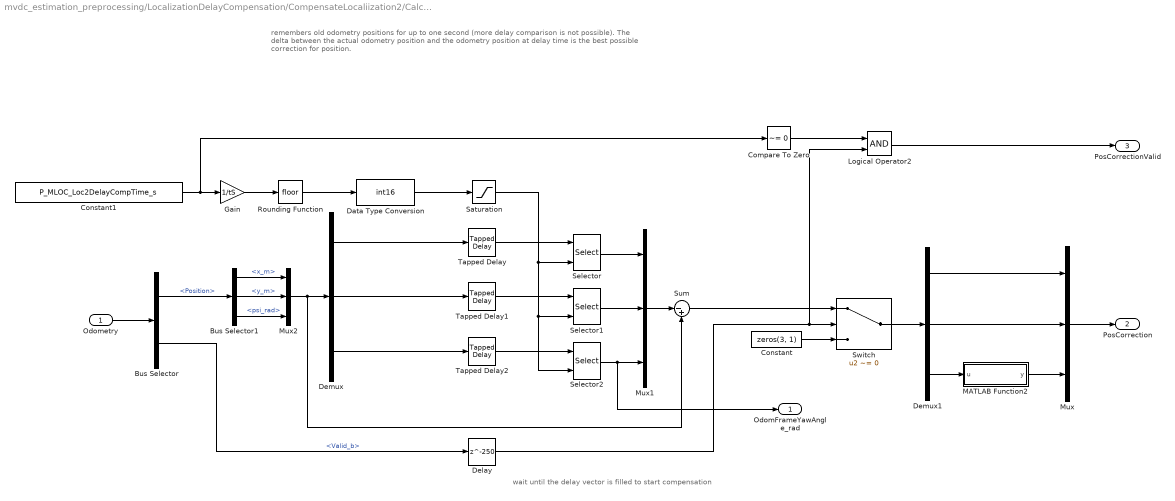
== system mvdc_estimation_preprocessing/LocalizationDelayCompensation/CompensateLocaliization2/CalculateDelayCompensation1 ==
  note: wait until the delay vector is filled to start compensation
  note: remembers old odometry positions for up to one second (more delay comparison is not possible).
      | The delta between the actual odometry position and the odometry position at delay time is the best possible correction for position.
  Odometry : Inport
  Bus Selector : BusSelector  OutputSignals=Position,Valid_b
  Bus Selector1 : BusSelector  OutputSignals=x_m,y_m,psi_rad
  Compare To Zero : simulink/Logic and Bit Operations/Compare To Zero  relop=~=  OutDataTypeStr=boolean
  Constant : Constant  Value=zeros(3, 1)
  Constant1 : Constant  Value=P_MLOC_Loc2DelayCompTime_s
  Data Type Conversion : DataTypeConversion  OutDataTypeStr=int16
  Delay : Delay  DelayLength=250
  Demux : Demux  Outputs=3
  Demux1 : Demux  Outputs=3
  Gain : Gain  Gain=1/tS
  Logical Operator2 : Logic  AllPortsSameDT=off  OutDataTypeStr=boolean
  MATLAB Function2 : MATLAB Function  TreatAsAtomicUnit=on
  Mux : Mux  Inputs=3
  Mux1 : Mux  Inputs=3
  Mux2 : Mux  Inputs=3
  Rounding Function : Rounding
  Saturation : Saturate  UpperLimit=249  LowerLimit=0
  Selector : Selector  IndexMode=Zero-based  InputPortWidth=250  IndexOptions=Index vector (port)  Indices=[1 3]  OutputSizes=1
  Selector1 : Selector  IndexMode=Zero-based  InputPortWidth=250  IndexOptions=Index vector (port)  Indices=[1 3]  OutputSizes=1
  Selector2 : Selector  IndexMode=Zero-based  InputPortWidth=250  IndexOptions=Index vector (port)  Indices=[1 3]  OutputSizes=1
  Sum : Sum  Inputs=|-+
  Switch : Switch  Criteria=u2 ~= 0  Threshold=249
  Tapped Delay : simulink/Discrete/Tapped Delay  vinit=0.0  samptime=-1  NumDelays=249  DelayOrder=Newest  includeCurrent=on
  Tapped Delay1 : simulink/Discrete/Tapped Delay  vinit=0.0  samptime=-1  NumDelays=249  DelayOrder=Newest  includeCurrent=on
  Tapped Delay2 : simulink/Discrete/Tapped Delay  vinit=0.0  samptime=-1  NumDelays=249  DelayOrder=Newest  includeCurrent=on
  OdomFrameYawAngle_rad : Outport
  PosCorrection : Outport  Port=2
  PosCorrectionValid : Outport  Port=3
  wires:
  Gain/1 -> Rounding Function/1
  Rounding Function/1 -> Data Type Conversion/1
  Data Type Conversion/1 -> Saturation/1
  Mux2/1 -> Sum/2, Demux/1
  Demux/1 -> Tapped Delay/1
  Demux/2 -> Tapped Delay1/1
  Demux/3 -> Tapped Delay2/1
  Mux/1 -> PosCorrection/1
  Demux1/2 -> Mux/2
  MATLAB Function2/1(y) -> Mux/3
  Mux1/1 -> Sum/1
  Selector/1 -> Mux1/1
  Selector2/1 -> OdomFrameYawAngle_rad/1, Mux1/3
  Selector1/1 -> Mux1/2
  Tapped Delay2/1 -> Selector2/1
  Tapped Delay1/1 -> Selector1/1
  Tapped Delay/1 -> Selector/1
  Demux1/3 -> MATLAB Function2/1(u)
  Switch/1 -> Demux1/1
  Sum/1 -> Switch/1
  Bus Selector/2 -> Delay/1  "<Valid_b>"
  Bus Selector/1 -> Bus Selector1/1  "<Position>"
  Odometry/1 -> Bus Selector/1
  Constant/1 -> Switch/3
  Delay/1 -> Logical Operator2/2, Switch/2
  Demux1/1 -> Mux/1
  Bus Selector1/1 -> Mux2/1  "<x_m>"
  Bus Selector1/2 -> Mux2/2  "<y_m>"
  Bus Selector1/3 -> Mux2/3  "<psi_rad>"
  Logical Operator2/1 -> PosCorrectionValid/1
  Constant1/1 -> Compare To Zero/1, Gain/1
  Compare To Zero/1 -> Logical Operator2/1
  Saturation/1 -> Selector2/2, Selector1/2, Selector/2

== system mvdc_estimation_preprocessing/LocalizationDelayCompensation/CompensateLocaliization2/RotateCompensation1 ==
  note: As the odometry is not necessarily aligned with the actual vehicle coordinates,
      | it is necessary to consider only the relative changes of the vehicle. Therefore
      | the calculated difference in x and y coordinates has to be transformed between
      | the odometry coordinate frame at the time instant where the pose measurement was taken
      | and added to the measured vehicle pose correctly.
  Orientation_LocFrame_rad : Inport
  Orientation_OdomFrame_rad : Inport  Port=2
  Comp_OdomFrame : Inport  Port=3
  Demux : Demux  Outputs=3
  MATLAB Function2 : MATLAB Function  TreatAsAtomicUnit=on
  Mux : Mux  Inputs=3
  RotationTransform : misc/RotationTransform  SystemSampleTime=-1
  RotationTransform1 : misc/RotationTransform  SystemSampleTime=-1
  Unary Minus : UnaryMinus
  Comp_MeasFrame : Outport
  wires:
  Unary Minus/1 -> RotationTransform/3
  RotationTransform/2 -> RotationTransform1/2
  RotationTransform/1 -> RotationTransform1/1
  Orientation_LocFrame_rad/1 -> RotationTransform1/3
  Orientation_OdomFrame_rad/1 -> Unary Minus/1
  Comp_OdomFrame/1 -> Demux/1
  Demux/1 -> RotationTransform/1
  Demux/2 -> RotationTransform/2
  Demux/3 -> MATLAB Function2/1(u)
  RotationTransform1/1 -> Mux/1
  RotationTransform1/2 -> Mux/2
  MATLAB Function2/1(y) -> Mux/3
  Mux/1 -> Comp_MeasFrame/1

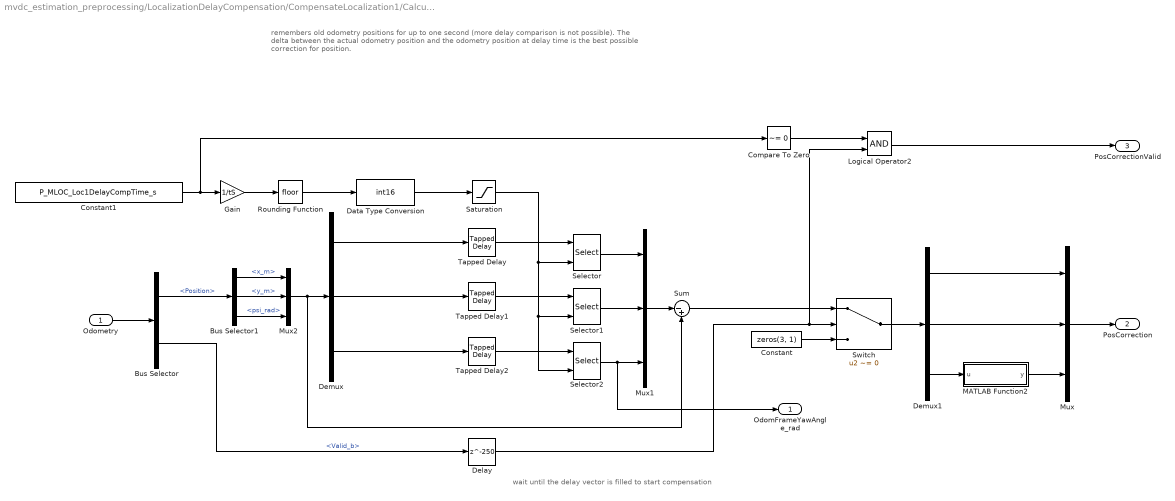
== system mvdc_estimation_preprocessing/LocalizationDelayCompensation/CompensateLocalization1/CalculateDelayCompensation1 ==
  note: wait until the delay vector is filled to start compensation
  note: remembers old odometry positions for up to one second (more delay comparison is not possible).
      | The delta between the actual odometry position and the odometry position at delay time is the best possible correction for position.
  Odometry : Inport
  Bus Selector : BusSelector  OutputSignals=Position,Valid_b
  Bus Selector1 : BusSelector  OutputSignals=x_m,y_m,psi_rad
  Compare To Zero : simulink/Logic and Bit Operations/Compare To Zero  relop=~=  OutDataTypeStr=boolean
  Constant : Constant  Value=zeros(3, 1)
  Constant1 : Constant  Value=P_MLOC_Loc1DelayCompTime_s
  Data Type Conversion : DataTypeConversion  OutDataTypeStr=int16
  Delay : Delay  DelayLength=250
  Demux : Demux  Outputs=3
  Demux1 : Demux  Outputs=3
  Gain : Gain  Gain=1/tS
  Logical Operator2 : Logic  AllPortsSameDT=off  OutDataTypeStr=boolean
  MATLAB Function2 : MATLAB Function  TreatAsAtomicUnit=on
  Mux : Mux  Inputs=3
  Mux1 : Mux  Inputs=3
  Mux2 : Mux  Inputs=3
  Rounding Function : Rounding
  Saturation : Saturate  UpperLimit=249  LowerLimit=0
  Selector : Selector  IndexMode=Zero-based  InputPortWidth=250  IndexOptions=Index vector (port)  Indices=[1 3]  OutputSizes=1
  Selector1 : Selector  IndexMode=Zero-based  InputPortWidth=250  IndexOptions=Index vector (port)  Indices=[1 3]  OutputSizes=1
  Selector2 : Selector  IndexMode=Zero-based  InputPortWidth=250  IndexOptions=Index vector (port)  Indices=[1 3]  OutputSizes=1
  Sum : Sum  Inputs=|-+
  Switch : Switch  Criteria=u2 ~= 0  Threshold=249
  Tapped Delay : simulink/Discrete/Tapped Delay  vinit=0.0  samptime=-1  NumDelays=249  DelayOrder=Newest  includeCurrent=on
  Tapped Delay1 : simulink/Discrete/Tapped Delay  vinit=0.0  samptime=-1  NumDelays=249  DelayOrder=Newest  includeCurrent=on
  Tapped Delay2 : simulink/Discrete/Tapped Delay  vinit=0.0  samptime=-1  NumDelays=249  DelayOrder=Newest  includeCurrent=on
  OdomFrameYawAngle_rad : Outport
  PosCorrection : Outport  Port=2
  PosCorrectionValid : Outport  Port=3
  wires:
  Gain/1 -> Rounding Function/1
  Rounding Function/1 -> Data Type Conversion/1
  Data Type Conversion/1 -> Saturation/1
  Mux2/1 -> Sum/2, Demux/1
  Demux/1 -> Tapped Delay/1
  Demux/2 -> Tapped Delay1/1
  Demux/3 -> Tapped Delay2/1
  Mux/1 -> PosCorrection/1
  Demux1/2 -> Mux/2
  MATLAB Function2/1(y) -> Mux/3
  Mux1/1 -> Sum/1
  Selector/1 -> Mux1/1
  Selector2/1 -> OdomFrameYawAngle_rad/1, Mux1/3
  Selector1/1 -> Mux1/2
  Tapped Delay2/1 -> Selector2/1
  Tapped Delay1/1 -> Selector1/1
  Tapped Delay/1 -> Selector/1
  Demux1/3 -> MATLAB Function2/1(u)
  Switch/1 -> Demux1/1
  Sum/1 -> Switch/1
  Bus Selector/2 -> Delay/1  "<Valid_b>"
  Bus Selector/1 -> Bus Selector1/1  "<Position>"
  Odometry/1 -> Bus Selector/1
  Constant/1 -> Switch/3
  Delay/1 -> Logical Operator2/2, Switch/2
  Demux1/1 -> Mux/1
  Bus Selector1/1 -> Mux2/1  "<x_m>"
  Bus Selector1/2 -> Mux2/2  "<y_m>"
  Bus Selector1/3 -> Mux2/3  "<psi_rad>"
  Logical Operator2/1 -> PosCorrectionValid/1
  Constant1/1 -> Compare To Zero/1, Gain/1
  Compare To Zero/1 -> Logical Operator2/1
  Saturation/1 -> Selector2/2, Selector1/2, Selector/2

== system mvdc_estimation_preprocessing/LocalizationDelayCompensation/CompensateLocalization1/RotateCompensation ==
  note: As the odometry is not necessarily aligned with the actual vehicle coordinates,
      | it is necessary to consider only the relative changes of the vehicle. Therefore
      | the calculated difference in x and y coordinates has to be transformed between
      | the odometry coordinate frame at the time instant where the pose measurement was taken
      | and added to the measured vehicle pose correctly.
  Orientation_LocFrame_rad : Inport
  Orientation_OdomFrame_rad : Inport  Port=2
  Comp_OdomFrame : Inport  Port=3
  Demux : Demux  Outputs=3
  MATLAB Function2 : MATLAB Function  TreatAsAtomicUnit=on
  Mux : Mux  Inputs=3
  RotationTransform : misc/RotationTransform  SystemSampleTime=-1
  RotationTransform1 : misc/RotationTransform  SystemSampleTime=-1
  Unary Minus : UnaryMinus
  Comp_MeasFrame : Outport
  wires:
  Unary Minus/1 -> RotationTransform/3
  RotationTransform/2 -> RotationTransform1/2
  RotationTransform/1 -> RotationTransform1/1
  Orientation_LocFrame_rad/1 -> RotationTransform1/3
  Orientation_OdomFrame_rad/1 -> Unary Minus/1
  Comp_OdomFrame/1 -> Demux/1
  Demux/1 -> RotationTransform/1
  Demux/2 -> RotationTransform/2
  Demux/3 -> MATLAB Function2/1(u)
  RotationTransform1/1 -> Mux/1
  RotationTransform1/2 -> Mux/2
  MATLAB Function2/1(y) -> Mux/3
  Mux/1 -> Comp_MeasFrame/1

== matlab function mvdc_estimation_preprocessing/LocalizationDelayCompensation/CompensateLocalization1/CalculateDelayCompensation1/MATLAB Function2 ==
  data: u input; y output
function y = fcn(u)

y = normalizeAngle(u);

== matlab function mvdc_estimation_preprocessing/CalculateOdometry/IntegrateOdometry/MATLAB Function ==
  data: vx_mps input; Position output Bus: CartPos; vy_mps input; dPsi_rad input; OdometryPosition_old input Bus: CartPos; tS parameter
function Position  = fcn_integrateOdometry(vx_mps, vy_mps, dPsi_rad, OdometryPosition_old, tS)

[Position] = integrateOdometry(vx_mps, vy_mps, dPsi_rad, OdometryPosition_old, tS);

== matlab function mvdc_estimation_preprocessing/LocalizationDelayCompensation/CompensateLocalization1/RotateCompensation/MATLAB Function2 ==
  data: u input; y output
function y = fcn(u)

y = normalizeAngle(u);

== matlab function mvdc_estimation_preprocessing/Diagnosis/ParseResidualsToFailedSensors/MATLAB Function ==
  data: resOK input boolean; FailureMode output boolean
function FailureMode = fcn(resOK)

% check if there is a failure
if sum(resOK) == 1
    FailureMode = resOK; 
else
    FailureMode = zeros(size(resOK), 'logical'); 
end

== matlab function mvdc_estimation_preprocessing/LocalizationDelayCompensation/CompensateLocaliization2/CalculateDelayCompensation1/MATLAB Function2 ==
  data: u input; y output
function y = fcn(u)

y = normalizeAngle(u);

== matlab function mvdc_estimation_preprocessing/Diagnosis/Truth Table1 ==
  data: valid_Loc1_b input boolean; valid_Loc2_b input boolean; valid_Vel1_b input boolean; valid_Vel2_b input boolean; valid_IMU1_b input boolean; valid_IMU2_b input boolean; valid_Wheelspeeds_b input boolean; SE_State output Enum: TUMStateEstimationState; SE_Status output Enum: TUMHealthStatus
function [SE_State, SE_Status] = fcn(valid_Loc1_b, valid_Loc2_b, valid_Vel1_b, valid_Vel2_b, valid_IMU1_b, valid_IMU2_b, valid_Wheelspeeds_b)

aVarTruthTableCondition_1 = false;
aVarTruthTableCondition_2 = false;
aVarTruthTableCondition_3 = false;
aVarTruthTableCondition_4 = false;


% Localization available

aVarTruthTableCondition_1 = logical(valid_Loc1_b || valid_Loc2_b);

% Velocity available

aVarTruthTableCondition_2 = logical(valid_Vel1_b || valid_Vel2_b);

% IMU available

aVarTruthTableCondition_3 = logical(valid_IMU1_b || valid_IMU2_b);

% Odometry speed source available

aVarTruthTableCondition_4 = logical(valid_Vel1_b  || valid_Vel2_b || valid_Wheelspeeds_b);

if (aVarTruthTableCondition_1 && aVarTruthTableCondition_3)
    aFcnTruthTableAction_1();
elseif (aVarTruthTableCondition_3 && aVarTruthTableCondition_4)
    aFcnTruthTableAction_2();
else % Default
    aFcnTruthTableAction_3();
end

function aFcnTruthTableAction_1()

% Sensor fusion using all configured sensors

SE_State = TUMStateEstimationState.SE_NORMAL
SE_Status = TUMHealthStatus.OK

function aFcnTruthTableAction_2()

% Sensor fusion not working, stop the car using standard emergency stop on odometry

SE_State = TUMStateEstimationState.SE_ODOM
SE_Status = TUMHealthStatus.WARNING

function aFcnTruthTableAction_3()

% Sensors are complete crap, stop the car using hard emergency stop

SE_State = TUMStateEstimationState.SE_FAIL
SE_Status = TUMHealthStatus.ERROR

== matlab function mvdc_estimation_preprocessing/LocalizationDelayCompensation/CompensateLocaliization2/RotateCompensation1/MATLAB Function2 ==
  data: u input; y output
function y = fcn(u)

y = normalizeAngle(u);
